simulink model "b2a_th2"  (R2018a)
settings: Solver=VariableStepAuto  StartTime=0.0  StopTime=100  RelTol=1e-3
libraries: simulink x1
settings Model: Creator=Huy  LastModifiedBy=Huy

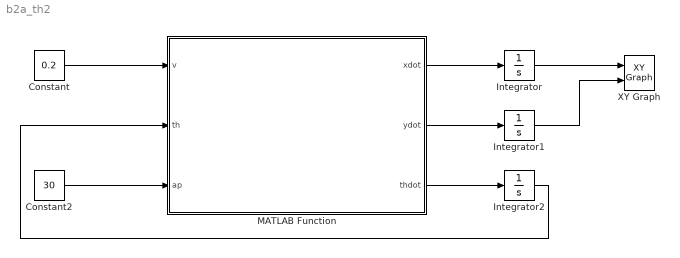
== system b2a_th2 ==
  Constant : Constant  Value=0.2
  Constant2 : Constant  Value=30
  Integrator : Integrator
  Integrator1 : Integrator
  Integrator2 : Integrator
  MATLAB Function : MATLAB Function  TreatAsAtomicUnit=on
  XY Graph : simulink/Sinks/XY Graph  xmin=-5  xmax=5  ymin=-5  ymax=5  st=1
  wires:
  MATLAB Function/1(xdot) -> Integrator/1
  Constant/1 -> MATLAB Function/1(v)
  Constant2/1 -> MATLAB Function/3(ap)
  MATLAB Function/2(ydot) -> Integrator1/1
  MATLAB Function/3(thdot) -> Integrator2/1
  Integrator/1 -> XY Graph/1
  Integrator1/1 -> XY Graph/2
  Integrator2/1 -> MATLAB Function/2(th)

== matlab function b2a_th2/MATLAB Function ==
  data: v input; xdot output; th input; ap input; ydot output; thdot output
function [xdot,ydot,thdot] = tricycle (v,th,ap)
vmax = 0.36; 
amax = 0.28;
apmax = (pi/4)*180/pi 
wmax = 0.30;  
G = 13;
d = sqrt(2.5 + 0.1*G);
xdot = v*cos(th);
ydot = v*sin(th);
thdot = v/d *sin(ap);
%vc = v/cos(alpha);
%vcmax=0.36/sqrt(2)/2=0.509m/s;                                
%vcmin = 0 m/s;
